simulink subsystem "Potentiometer2_SubSystem"  (R2020b)
settings: Solver=VariableStepAuto  StartTime=0.0  StopTime=10.0  RelTol=1e-3
values from neighbouring files (symbols this model uses):
  Ts = 0.001    [loadParNominalHubBeam.m]
undefined symbols (not defined in the file or in its folder): sens
settings Model: Creator=umberto  LastModifiedBy=umberto

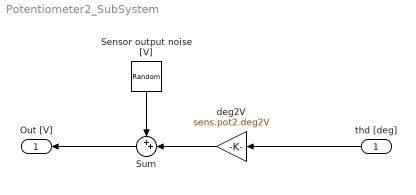
== system Potentiometer2_SubSystem ==
  thd [deg] : Inport
  Sensor output noise [V] : RandomNumber  Variance=sens.pot2.noise.var  SampleTime=Ts
  Sum : Sum  Inputs=++|
  deg2V : Gain  Gain=sens.pot2.deg2V
  Out [V] : Outport
  wires:
  Sum/1 -> Out [V]/1
  Sensor output noise [V]/1 -> Sum/1
  deg2V/1 -> Sum/2
  thd [deg]/1 -> deg2V/1
